simulink model "ego0_gap_not_desired"  (R2025b)
settings: Solver=VariableStepAuto  StartTime=0.0  StopTime=10.0  RelTol=1e-3
settings Model: Creator=jdcjd  LastModifiedBy=jdcjd

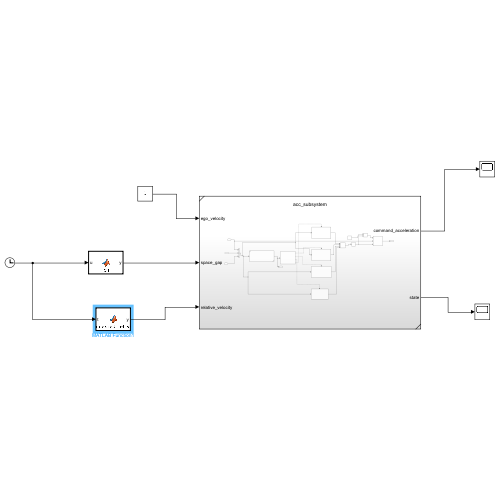
[thumbnail: Simulink's stored preview of the top-level diagram]
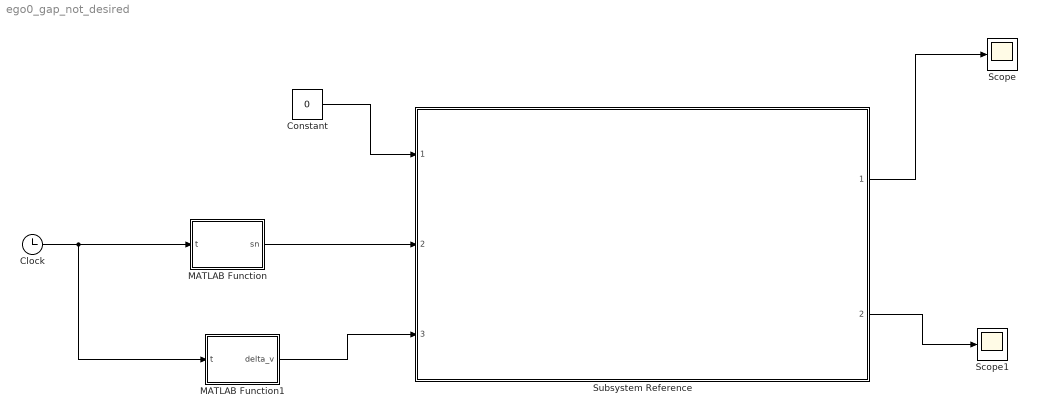
== system ego0_gap_not_desired ==
  Clock : Clock
  Constant : Constant  Value=0
  MATLAB Function : MATLAB Function  TreatAsAtomicUnit=on
  MATLAB Function1 : MATLAB Function  TreatAsAtomicUnit=on
  Scope : Scope
  Scope1 : Scope
  Subsystem Reference : Subsystem  ReferencedSubsystem=acc_subsystem
  wires:
  Subsystem Reference/2 -> Scope1/1
  Subsystem Reference/1 -> Scope/1
  Constant/1 -> Subsystem Reference/1
  MATLAB Function/1(sn) -> Subsystem Reference/2
  Clock/1 -> MATLAB Function1/1(t), MATLAB Function/1(t)
  MATLAB Function1/1(delta_v) -> Subsystem Reference/3

== matlab function ego0_gap_not_desired/MATLAB Function ==
  data: t input; sn output
function sn = undesired_sn(t)

sn = min(t, 0.9);
end

== matlab function ego0_gap_not_desired/MATLAB Function1 ==
  data: t input; delta_v output
function delta_v = undesired_rel_vel(t)

delta_v = min(t, 5)
